simulink model "EV3_rotation"  (R2025b)
settings: Solver=VariableStepAuto  StartTime=0.0  StopTime=10.0  RelTol=1e-3
values from neighbouring files (symbols this model uses):
  K1 = lqrd(A1,B1,C1'*C1,0.01,Ts)    [model_discret.m]
  K2 = A2(2,2)^2/(4*B2(2,1))    [model_discret.m]
  R = 0.027    [model.m]
  Ts = 0.004    [model.m]
  W = 0.085    [model.m]
undefined symbols (not defined in the file or in its folder): DiscIntNeverNeededParam, gamma, K_PWM
libraries: legoev3lib x5, simulink x1
settings Model: Creator=carol  LastModifiedBy=alber

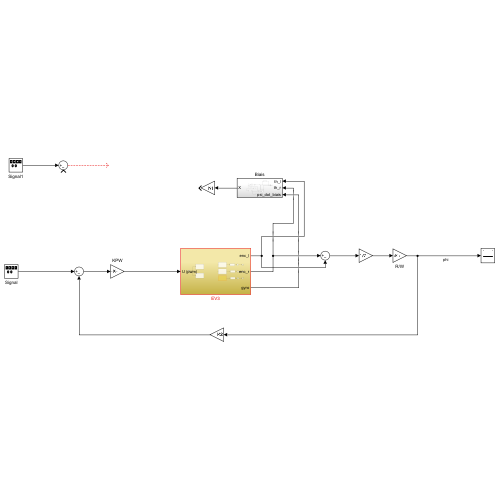
[thumbnail: Simulink's stored preview of the top-level diagram]
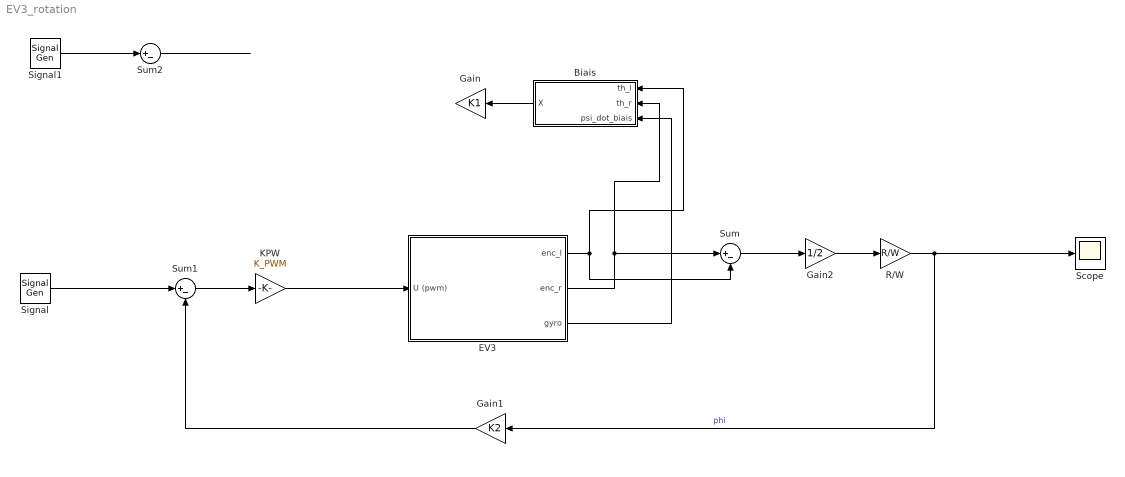
== system EV3_rotation ==
  Biais : Subsystem
  EV3 : Subsystem
  Gain : Gain  Gain=K1
  Gain1 : Gain  Gain=K2
  Gain2 : Gain  Gain=1/2
  KPW : Gain  Gain=K_PWM
  R/W : Gain  Gain=R/W
  Scope : Scope
  Signal : SignalGenerator  WaveForm=square  Amplitude=0  Frequency=0.1
  Signal1 : SignalGenerator  WaveForm=square  Amplitude=0  Frequency=0.1
  Sum : Sum  Inputs=|+-
  Sum1 : Sum  Inputs=|+-
  Sum2 : Sum  Inputs=|+-
  wires:
  EV3/2(enc_r) -> Biais/2(th_r), Sum/1
  Sum/1 -> Gain2/1
  Gain2/1 -> R/W/1
  EV3/1(enc_l) -> Biais/1(th_l), Sum/2
  R/W/1 -> Scope/1, Gain1/1  "phi"
  Gain1/1 -> Sum1/2
  Sum1/1 -> KPW/1
  KPW/1 -> EV3/1(U (pwm))
  Signal/1 -> Sum1/1
  Biais/1(X) -> Gain/1
  Sum2/1 -> ?
  Signal1/1 -> Sum2/1
  EV3/3(gyro) -> Biais/3(psi_dot_biais)

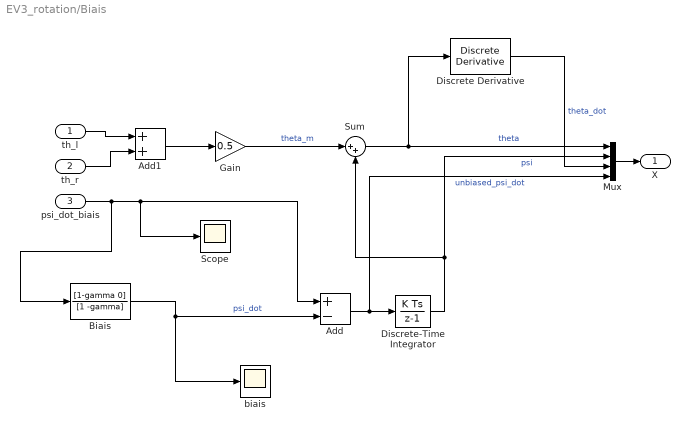
== system EV3_rotation/Biais ==
  th_l : Inport
  th_r : Inport  Port=2
  psi_dot_biais : Inport  Port=3
  Add : Sum  Inputs=+-
  Add1 : Sum
  Biais : DiscreteTransferFcn  Numerator=[1-gamma 0]  Denominator=[1 -gamma]
  Discrete Derivative : simulink/Quick Insert/Discrete/Discrete Derivative  gainval=1.0  ICPrevScaledInput=0.0  OutMin=[]  OutMax=[]  OutDataType=fixdt(1, 16)  OutScaling=2^-10  DoSatur=off
  Discrete-Time Integrator : DiscreteIntegrator  SampleTime=Ts  ICPrevOutput=DiscIntNeverNeededParam  ICPrevScaledInput=DiscIntNeverNeededParam
  Gain : Gain  Gain=0.5
  Mux : Mux
  Scope : Scope
      settings: ActiveDisplayYMinimum=-1  ActiveDisplayYMaximum=1  DataLoggingVariableName=ScopeData13
  Sum : Sum  Inputs=|++
  biais : Scope
      settings: ActiveDisplayYMinimum=-0.1164059395354744  ActiveDisplayYMaximum=0.0646369691442869  DataLoggingVariableName=ScopeData12
  X : Outport
  wires:
  th_l/1 -> Add1/1
  th_r/1 -> Add1/2
  Add1/1 -> Gain/1
  Mux/1 -> X/1
  Discrete Derivative/1 -> Mux/3  "theta_dot"
  Discrete-Time Integrator/1 -> Sum/2, Mux/2  "psi"
  psi_dot_biais/1 -> Biais/1, Scope/1, Add/1
  Biais/1 -> Add/2, biais/1  "psi_dot"
  Add/1 -> Mux/4, Discrete-Time Integrator/1  "unbiased_psi_dot"
  Gain/1 -> Sum/1  "theta_m"
  Sum/1 -> Mux/1, Discrete Derivative/1  "theta"

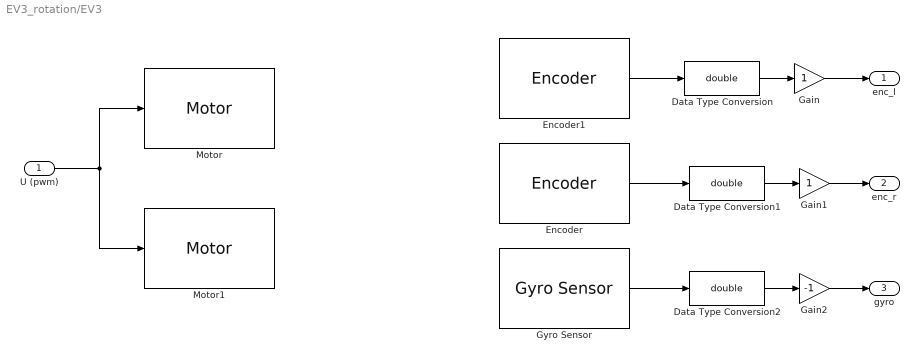
== system EV3_rotation/EV3 ==
  U (pwm) : Inport
  Data Type Conversion : DataTypeConversion  OutDataTypeStr=double  SaturateOnIntegerOverflow=off  RndMeth=Floor
  Data Type Conversion1 : DataTypeConversion  OutDataTypeStr=double  SaturateOnIntegerOverflow=off  RndMeth=Floor
  Data Type Conversion2 : DataTypeConversion  OutDataTypeStr=double  SaturateOnIntegerOverflow=off  RndMeth=Floor
  Encoder : legoev3lib/Encoder  portNumber=A  opMode=Reset by external signal  sampleTime=Ts
  Encoder1 : legoev3lib/Encoder  portNumber=D  opMode=Reset by external signal  sampleTime=Ts
  Gain : Gain
  Gain1 : Gain
  Gain2 : Gain  Gain=-1
  Gyro Sensor : legoev3lib/Gyro Sensor  portNumber=3  sampleTime=Ts
  Motor : legoev3lib/Motor  sportNumber=D  sstopAction=Brake
  Motor1 : legoev3lib/Motor  sportNumber=A  sstopAction=Brake
  enc_l : Outport
  enc_r : Outport  Port=2
  gyro : Outport  Port=3
  wires:
  Gyro Sensor/1 -> Data Type Conversion2/1
  Encoder/1 -> Data Type Conversion1/1
  Encoder1/1 -> Data Type Conversion/1
  Data Type Conversion/1 -> Gain/1
  Data Type Conversion1/1 -> Gain1/1
  Data Type Conversion2/1 -> Gain2/1
  U (pwm)/1 -> Motor1/1, Motor/1
  Gain/1 -> enc_l/1
  Gain1/1 -> enc_r/1
  Gain2/1 -> gyro/1
